simulink model "BS_ur10v"  (R2021b)
settings: Solver=VariableStepAuto  StartTime=0.0  StopTime=15.0  RelTol=1e-3
undefined symbols (not defined in the file): Kd, l1, l2, l3, l4, l5, l6, lambda, m1, m2, m3, m4, m5, m6, q0, r
libraries: roblocks x3
(part 1 of 3)
settings Model: Creator=pierg  LastModifiedBy=vince

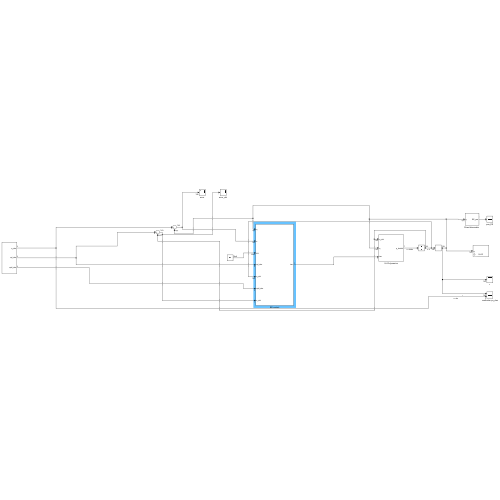
[thumbnail: Simulink's stored preview of the top-level diagram]
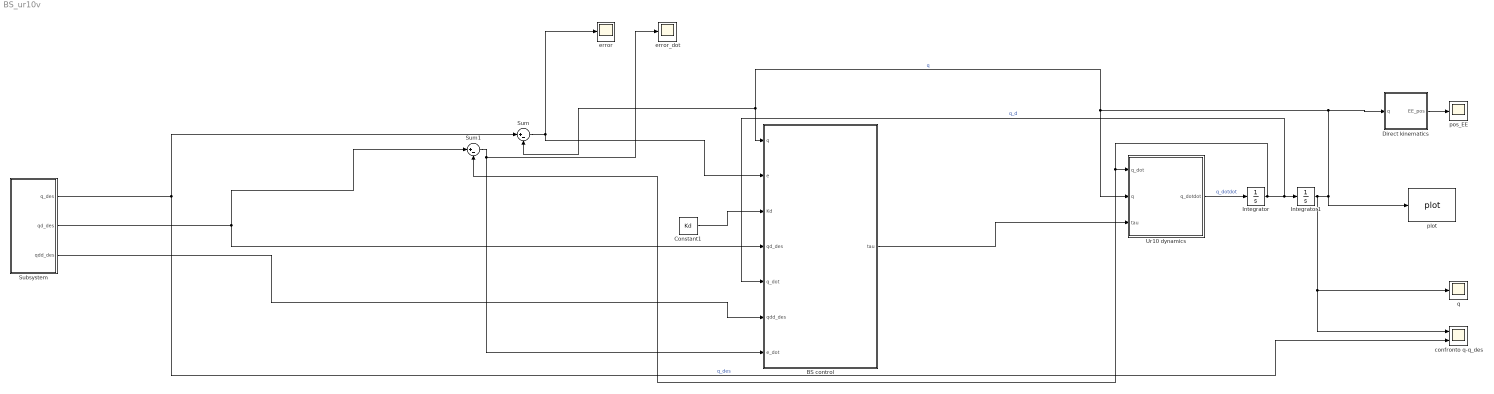
== system BS_ur10v ==
  BS control : Subsystem
  Constant1 : Constant  Value=Kd
  Direct kinematics : Subsystem
  Integrator : Integrator  InitialCondition=[0.001 0.001 0.001 0.001 0.001 0.001]'
  Integrator1 : Integrator  InitialCondition=q0'
  Subsystem : Subsystem
  Sum : Sum  Inputs=|+-
  Sum1 : Sum  Inputs=|+-
  Ur10 dynamics : Subsystem
  confronto q-q_des : Scope  NumInputPorts=2
  error : Scope
  error_dot : Scope
  plot : roblocks/Arm/plot  robot=ur10  fps=20  holdplot=on
  pos_EE : Scope
  q : Scope
  wires:
  Ur10 dynamics/1(q_dotdot) -> Integrator/1  "q_dotdot"
  Integrator/1 -> Ur10 dynamics/1(q_dot), Sum1/2, BS control/5(q_dot), Integrator1/1  "q_d"
  BS control/1(tau) -> Ur10 dynamics/3(tau)
  Integrator1/1 -> confronto q-q_des/1, q/1, plot/1, Direct kinematics/1(q), Ur10 dynamics/2(q), Sum/2, BS control/1(q)  "q"
  Constant1/1 -> BS control/3(Kd)
  Subsystem/1(q_des) -> Sum/1, confronto q-q_des/2  "q_des"
  Subsystem/2(qd_des) -> BS control/4(qd_des), Sum1/1
  Sum/1 -> error/1, BS control/2(e)
  Sum1/1 -> BS control/7(e_dot), error_dot/1
  Direct kinematics/1(EE_pos) -> pos_EE/1
  Subsystem/3(qdd_des) -> BS control/6(qdd_des)

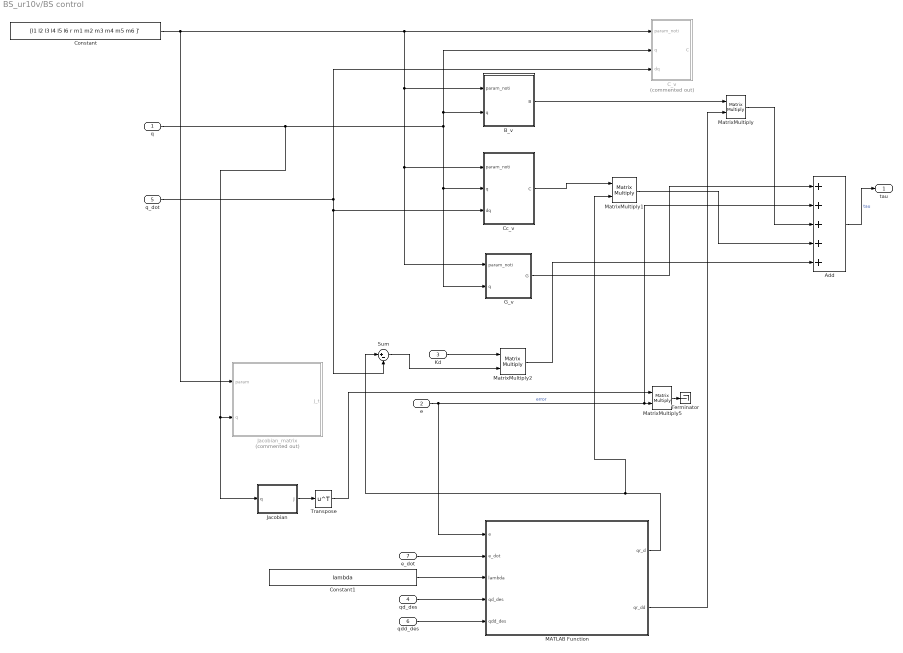
== system BS_ur10v/BS control ==
  q : Inport
  e : Inport  Port=2
  Kd : Inport  Port=3
  qd_des : Inport  Port=4
  q_dot : Inport  Port=5
  qdd_des : Inport  Port=6
  e_dot : Inport  Port=7
  Add : Sum  Inputs=+++++
  B_v : MATLAB Function  TreatAsAtomicUnit=on
  C_v : MATLAB Function  Commented=on  TreatAsAtomicUnit=on
  Cc_v : MATLAB Function  TreatAsAtomicUnit=on
  Constant : Constant  Value=[l1 l2 l3 l4 l5 l6 r m1 m2 m3 m4 m5 m6 ]'
  Constant1 : Constant  Value=lambda
  G_v : MATLAB Function  TreatAsAtomicUnit=on
  Jacobian : MATLAB Function  TreatAsAtomicUnit=on
  Jacobian_matrix : MATLAB Function  Commented=on  TreatAsAtomicUnit=on
  MATLAB Function : MATLAB Function  TreatAsAtomicUnit=on
  MatrixMultiply{,1..2,5} (4 alike) : Product  Multiplication=Matrix(*)
  Sum : Sum  Inputs=|+-
  Terminator : Terminator
  Transpose : Math  Operator=transpose  SaturateOnIntegerOverflow=on
  tau : Outport
  wires:
  Add/1 -> tau/1  "tau"
  B_v/1(B) -> MatrixMultiply/1
  q/1 -> Jacobian_matrix/2(q), Jacobian/1(q), C_v/2(q), B_v/2(q), G_v/2(q), Cc_v/2(q)
  e/1 -> Add/2, MatrixMultiply5/2, MATLAB Function/1(e)  "error"
  MatrixMultiply1/1 -> Add/4
  MatrixMultiply/1 -> Add/3
  G_v/1(G) -> Add/1
  Kd/1 -> MatrixMultiply2/1
  Sum/1 -> MatrixMultiply2/2
  Constant1/1 -> MATLAB Function/3(lambda)
  Constant/1 -> Jacobian_matrix/1(param), G_v/1(param_noti), Cc_v/1(param_noti), B_v/1(param_noti), C_v/1(param_noti)
  qd_des/1 -> MATLAB Function/4(qd_des)
  MATLAB Function/1(qr_d) -> Sum/1, MatrixMultiply1/2
  q_dot/1 -> Sum/2, Cc_v/3(dq), C_v/3(dq)
  MatrixMultiply2/1 -> Add/5
  qdd_des/1 -> MATLAB Function/5(qdd_des)
  e_dot/1 -> MATLAB Function/2(e_dot)
  MATLAB Function/2(qr_dd) -> MatrixMultiply/2
  Jacobian/1(J) -> Transpose/1
  Transpose/1 -> MatrixMultiply5/1
  Cc_v/1(C) -> MatrixMultiply1/1
  MatrixMultiply5/1 -> Terminator/1

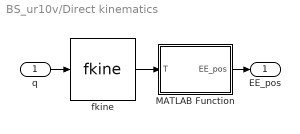
== system BS_ur10v/Direct kinematics ==
  q : Inport
  MATLAB Function : MATLAB Function  TreatAsAtomicUnit=on
  fkine : roblocks/Arm/fkine  robot=ur10
  EE_pos : Outport
  wires:
  q/1 -> fkine/1
  MATLAB Function/1(EE_pos) -> EE_pos/1
  fkine/1 -> MATLAB Function/1(T)

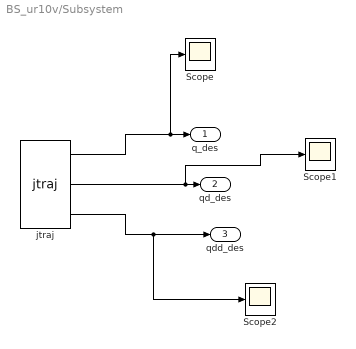
== system BS_ur10v/Subsystem ==
  Scope : Scope
  Scope1 : Scope
  Scope2 : Scope
  jtraj : roblocks/Toolbox/jtraj  q0=q0  qf=q_des_fin  tmax=15  ts=0.1
  q_des : Outport
  qd_des : Outport  Port=2
  qdd_des : Outport  Port=3
  wires:
  jtraj/2 -> Scope1/1, qd_des/1
  jtraj/3 -> qdd_des/1, Scope2/1
  jtraj/1 -> Scope/1, q_des/1

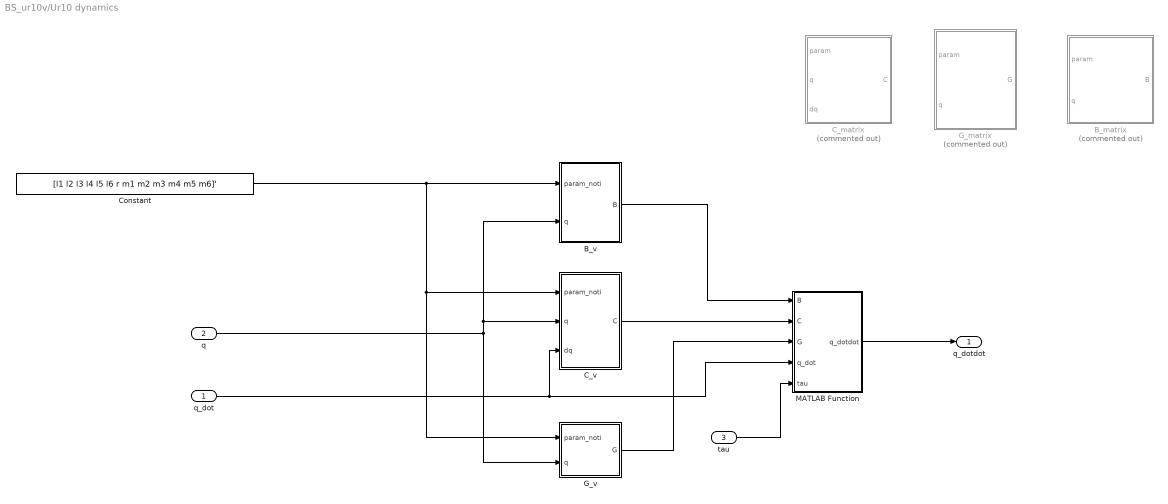
== system BS_ur10v/Ur10 dynamics ==
  q_dot : Inport
  q : Inport  Port=2
  tau : Inport  Port=3
  B_matrix : MATLAB Function  Commented=on  TreatAsAtomicUnit=on
  B_v : MATLAB Function  TreatAsAtomicUnit=on
  C_matrix : MATLAB Function  Commented=on  TreatAsAtomicUnit=on
  C_v : MATLAB Function  TreatAsAtomicUnit=on
  Constant : Constant  Value=[l1 l2 l3 l4 l5 l6 r m1 m2 m3 m4 m5 m6]'
  G_matrix : MATLAB Function  Commented=on  TreatAsAtomicUnit=on
  G_v : MATLAB Function  TreatAsAtomicUnit=on
  MATLAB Function : MATLAB Function  TreatAsAtomicUnit=on
  q_dotdot : Outport
  wires:
  Constant/1 -> G_v/1(param_noti), C_v/1(param_noti), B_v/1(param_noti)
  q/1 -> B_v/2(q), C_v/2(q), G_v/2(q)
  MATLAB Function/1(q_dotdot) -> q_dotdot/1
  q_dot/1 -> C_v/3(dq), MATLAB Function/4(q_dot)
  tau/1 -> MATLAB Function/5(tau)
  B_v/1(B) -> MATLAB Function/1(B)
  C_v/1(C) -> MATLAB Function/2(C)
  G_v/1(G) -> MATLAB Function/3(G)

== matlab function BS_ur10v/Ur10 dynamics/MATLAB Function ==
  data: B input; q_dotdot output; C input; G input; q_dot input; tau input
function q_dotdot = dynamics(B, C, G, q_dot, tau)
% Calcolo l'accelerazione dei giunti
q_dotdot = B \ (tau - C*q_dot - G);

== matlab function BS_ur10v/BS control/Jacobian ==
  data: q input; J output
function J = Jacobian(q)

q1 = q(1);
q2 = q(2);
q3 = q(3);
q4 = q(4);
q5 = q(5);
q6 = q(6);
%#codegen

%    This function was generated by the Symbolic Math Toolbox version 9.0.
%    01-Oct-2022 19:35:43

t2 = cos(q1);
t3 = cos(q2);
t4 = cos(q3);
t5 = cos(q4);
t6 = cos(q5);
t7 = sin(q1);
t8 = sin(q2);
t9 = sin(q3);
t10 = sin(q4);
t11 = sin(q5);
t12 = q2+q3;
t16 = -q5;
t13 = cos(t12);
t14 = q4+t12;
t15 = sin(t12);
t20 = -t2;
t24 = t8.*(1.53e+2./2.5e+2);
t17 = cos(t14);
t18 = q5+t14;
t19 = sin(t14);
t22 = t14+t16;
t25 = t13.*5.723e-1;
t26 = t15.*5.723e-1;
t27 = t10.*t13.*9.22e-2;
t28 = t5.*t15.*9.22e-2;
t34 = t5.*t13.*1.157e-1;
t36 = t10.*t15.*1.157e-1;
t21 = sin(t18);
t23 = sin(t22);
t29 = -t25;
t30 = t11.*t19.*9.22e-2;
t31 = t17.*1.157e-1;
t32 = t19.*1.157e-1;
t37 = -t36;
t39 = t27+t28;
t33 = t21.*4.61e-2;
t38 = t23.*4.61e-2;
t40 = t30+t31;
t41 = t11.*t39;
t35 = -t33;
t42 = t26+t40;
t43 = t24+t26+t34+t37+t41;
mt1 = [t2.*1.639e-1+t2.*t6.*9.22e-2+t3.*t7.*(1.53e+2./2.5e+2)+t3.*t4.*t7.*5.723e-1-t7.*t8.*t9.*5.723e-1-t5.*t7.*t15.*1.157e-1-t7.*t10.*t13.*1.157e-1+t7.*t11.*t17.*9.22e-2];
mt2 = [t7.*1.639e-1-t2.*t3.*(1.53e+2./2.5e+2)+t6.*t7.*9.22e-2-t2.*t3.*t4.*5.723e-1+t2.*t8.*t9.*5.723e-1+t2.*t5.*t15.*1.157e-1+t2.*t10.*t13.*1.157e-1-t2.*t11.*t17.*9.22e-2,0.0,0.0,0.0,1.0,t2.*t43,t7.*t43,t3.*(-1.53e+2./2.5e+2)+t29+t32+t35+t38,t7,t20,0.0,t2.*t42,t7.*t42,t29+t32+t35+t38,t7,t20,0.0,t2.*t40,t7.*t40,t32+t35+t38,t7,t20,0.0];
mt3 = [t7.*t11.*(-9.22e-2)-t2.*t3.*t4.*t5.*t6.*9.22e-2+t2.*t3.*t6.*t9.*t10.*9.22e-2+t2.*t4.*t6.*t8.*t10.*9.22e-2+t2.*t5.*t6.*t8.*t9.*9.22e-2,t2.*t11.*9.22e-2-t3.*t4.*t5.*t6.*t7.*9.22e-2+t3.*t6.*t7.*t9.*t10.*9.22e-2+t4.*t6.*t7.*t8.*t10.*9.22e-2+t5.*t6.*t7.*t8.*t9.*9.22e-2,t35-t38,t2.*t19,t7.*t19,-t17,0.0,0.0,0.0,t6.*t7+t11.*t17.*t20,t6.*t20-t7.*t11.*t17,-t11.*t19];
J = reshape([mt1,mt2,mt3],6,6);

== matlab function BS_ur10v/BS control/MATLAB Function ==
  data: e input; qr_d output; e_dot input; lambda input; qd_des input; qdd_des input; qr_dd output
function [qr_d , qr_dd]= qr_d_calculus(e,e_dot,lambda,qd_des,qdd_des)

qr_d = qd_des + lambda*e;

qr_dd = qdd_des + lambda*e_dot;


end

== matlab function BS_ur10v/Ur10 dynamics/C_v ==
  data: param_noti input; C output; q input; dq input
function C = C_v(param_noti, q, dq)
%#codegen
l1 = param_noti(1);
l2 = param_noti(2);
l3 = param_noti(3);
l4 = param_noti(4);
l5 = param_noti(5);
l6 = param_noti(6);
r  = param_noti(7);

m1 = param_noti(8);
m2 = param_noti(9);
m3 = param_noti(10);
m4 = param_noti(11);
m5 = param_noti(12);
m6 = param_noti(13);


q1 = q(1);
q2 = q(2);
q3 = q(3);
q4 = q(4);
q5 = q(5);
q6 = q(6);

dq1 = dq(1);
dq2 = dq(2);
dq3 = dq(3);
dq4 = dq(4);
dq5 = dq(5);
dq6 = dq(6);

%    This function was generated by the Symbolic Math Toolbox version 9.0.
%    24-Sep-2022 17:47:23

t2 = cos(q2);
t3 = cos(q3);
t4 = cos(q4);
t5 = cos(q5);
t6 = sin(q3);
t7 = sin(q4);
t8 = sin(q5);
t9 = q2+q3;
t10 = q2+q5;
t11 = q3+q4;
t12 = q4+q5;
t13 = l2.^2;
t14 = l3.^2;
t15 = l4.^2;
t16 = l5.^2;
t17 = l6.^2;
t18 = q2.*2.0;
t19 = q3.*2.0;
t20 = q4.*2.0;
t21 = q5.*2.0;
t22 = r.^2;
t32 = -q5;
t23 = sin(t18);
t24 = sin(t21);
t25 = cos(t9);
t26 = cos(t10);
t27 = cos(t11);
t28 = cos(t12);
t29 = q4+t9;
t30 = q5+t9;
t31 = q5+t11;
t33 = -t21;
t36 = t9+t12;
t38 = q2+t9;
t42 = q2+t32;
t43 = q4+t32;
t44 = t9.*2.0;
t47 = t9+t32;
t48 = t11+t32;
t50 = l3.*l5.*m6.*t4.*2.0;
t53 = dq2.*l3.*l5.*m6.*t4;
t54 = dq3.*l3.*l5.*m6.*t4;
t55 = dq4.*l3.*l5.*m6.*t4;
t56 = dq2.*l2.*l3.*m3.*t6;
t57 = dq2.*l2.*l3.*m4.*t6;
t58 = dq2.*l2.*l3.*m6.*t6;
t59 = dq1.*l4.*l6.*m6.*t8;
t60 = dq5.*l5.*l6.*m6.*t8;
t69 = l2.*l5.*m6.*t3.*t4.*2.0;
t70 = l3.*l6.*m6.*t4.*t5.*2.0;
t71 = l2.*l5.*m6.*t6.*t7.*2.0;
t72 = l3.*l6.*m6.*t7.*t8.*2.0;
t77 = dq2.*l2.*l5.*m6.*t3.*t4;
t78 = dq5.*l3.*l6.*m6.*t4.*t5;
t79 = dq2.*l2.*l5.*m6.*t6.*t7;
t80 = dq2.*l3.*l6.*m6.*t7.*t8;
t81 = dq3.*l3.*l6.*m6.*t7.*t8;
t82 = dq4.*l3.*l6.*m6.*t7.*t8;
t94 = (dq1.*l3.*l5.*m6.*t4)./2.0;
t96 = (dq1.*l2.*l3.*m3.*t6)./2.0;
t97 = (dq1.*l2.*l3.*m4.*t6)./2.0;
t98 = (dq1.*l2.*l3.*m6.*t6)./2.0;
t102 = l2.*l6.*m6.*t3.*t7.*t8.*2.0;
t103 = l2.*l6.*m6.*t4.*t6.*t8.*2.0;
t107 = dq2.*l2.*l6.*m6.*t3.*t7.*t8;
t108 = dq2.*l2.*l6.*m6.*t4.*t6.*t8;
t117 = (dq2.*m6.*t8.*t22)./4.0;
t118 = (dq3.*m6.*t8.*t22)./4.0;
t119 = (dq4.*m6.*t8.*t22)./4.0;
t120 = (dq5.*m6.*t8.*t22)./4.0;
t121 = (dq6.*m6.*t8.*t22)./4.0;
t126 = (m5.*t5.*t8.*t16)./6.0;
t128 = (m5.*t5.*t8.*t22)./2.0;
t129 = (m6.*t5.*t8.*t22)./2.0;
t157 = m6.*t5.*t8.*t17.*(1.3e+1./6.0);
t34 = cos(t30);
t35 = cos(t31);
t37 = sin(t29);
t39 = q2+t29;
t40 = sin(t38);
t41 = sin(t36);
t45 = cos(t42);
t46 = cos(t43);
t51 = t12+t30;
t52 = t10+t29;
t61 = t9+t29;
t62 = sin(t44);
t63 = cos(t47);
t64 = cos(t48);
t65 = t29+t32;
t66 = t29+t33;
t73 = dq2.*l3.*l4.*m4.*t25;
t74 = dq3.*l3.*l4.*m4.*t25;
t75 = dq2.*l3.*l4.*m6.*t25;
t76 = dq3.*l3.*l4.*m6.*t25;
t84 = -t53;
t85 = -t54;
t86 = t9+t36;
t93 = t20+t44;
t104 = t29+t36;
t113 = -t77;
t114 = -t78;
t115 = -t80;
t116 = -t81;
t125 = t29+t47;
t131 = (dq1.*l2.*l5.*m6.*t27)./2.0;
t132 = (dq1.*l2.*l6.*m6.*t26)./2.0;
t133 = (dq2.*l2.*l6.*m6.*t26)./2.0;
t134 = (dq2.*l3.*l6.*m6.*t28)./2.0;
t135 = (dq5.*l2.*l6.*m6.*t26)./2.0;
t136 = (dq1.*l3.*l6.*m6.*t28)./4.0;
t137 = (dq3.*l3.*l6.*m6.*t28)./2.0;
t138 = (dq4.*l3.*l6.*m6.*t28)./2.0;
t139 = (dq5.*l3.*l6.*m6.*t28)./2.0;
t141 = -t120;
t142 = -t121;
t152 = (dq1.*m2.*t13.*t23)./2.0;
t153 = (dq1.*m3.*t13.*t23)./2.0;
t154 = (dq1.*m4.*t13.*t23)./2.0;
t155 = (dq1.*m6.*t13.*t23)./2.0;
t156 = -t126;
t158 = t36.*2.0;
t160 = -t107;
t161 = -t108;
t181 = (dq2.*m5.*t16.*t24)./2.4e+1;
t182 = (dq3.*m5.*t16.*t24)./2.4e+1;
t183 = (dq4.*m5.*t16.*t24)./2.4e+1;
t184 = (dq5.*m5.*t16.*t24)./2.4e+1;
t185 = (dq1.*m5.*t16.*t24)./4.8e+1;
t186 = (dq2.*m5.*t22.*t24)./8.0;
t187 = (dq2.*m6.*t22.*t24)./8.0;
t188 = (dq3.*m5.*t22.*t24)./8.0;
t189 = (dq3.*m6.*t22.*t24)./8.0;
t190 = (dq4.*m5.*t22.*t24)./8.0;
t191 = (dq4.*m6.*t22.*t24)./8.0;
t192 = (dq5.*m5.*t22.*t24)./8.0;
t193 = (dq5.*m6.*t22.*t24)./8.0;
t194 = (dq1.*m5.*t22.*t24)./1.6e+1;
t195 = (dq1.*m6.*t22.*t24)./1.6e+1;
t196 = -t157;
t237 = dq2.*m6.*t17.*t24.*(1.3e+1./2.4e+1);
t238 = dq3.*m6.*t17.*t24.*(1.3e+1./2.4e+1);
t239 = dq4.*m6.*t17.*t24.*(1.3e+1./2.4e+1);
t240 = dq5.*m6.*t17.*t24.*(1.3e+1./2.4e+1);
t241 = dq1.*m6.*t17.*t24.*(1.3e+1./4.8e+1);
t49 = cos(t39);
t67 = cos(t52);
t68 = sin(t51);
t83 = cos(t61);
t87 = sin(t65);
t88 = sin(t66);
t89 = dq2.*l4.*l5.*m6.*t37;
t90 = dq3.*l4.*l5.*m6.*t37;
t91 = dq4.*l4.*l5.*m6.*t37;
t92 = cos(t86);
t95 = t32+t39;
t99 = dq1.*l2.*l3.*m3.*t40;
t100 = dq1.*l2.*l3.*m4.*t40;
t101 = dq1.*l2.*l3.*m6.*t40;
t105 = sin(t93);
t109 = -t73;
t110 = -t74;
t111 = -t75;
t112 = -t76;
t140 = sin(t104);
t143 = (dq1.*l3.*l6.*m6.*t34)./2.0;
t144 = (dq2.*l3.*l6.*m6.*t34)./2.0;
t145 = (dq2.*l2.*l6.*m6.*t35)./2.0;
t146 = (dq3.*l3.*l6.*m6.*t34)./2.0;
t147 = (dq1.*l2.*l6.*m6.*t35)./4.0;
t148 = (dq3.*l2.*l6.*m6.*t35)./2.0;
t149 = (dq4.*l2.*l6.*m6.*t35)./2.0;
t150 = (dq5.*l3.*l6.*m6.*t34)./2.0;
t151 = (dq5.*l2.*l6.*m6.*t35)./2.0;
t159 = cos(t125);
t162 = -t131;
t163 = -t134;
t164 = -t136;
t165 = -t137;
t166 = -t138;
t167 = -t139;
t168 = sin(t158);
t197 = (dq1.*l5.*l6.*m6.*t41)./2.0;
t198 = (dq2.*l4.*l6.*m6.*t41)./2.0;
t199 = (dq2.*l5.*l6.*m6.*t41)./2.0;
t200 = (dq3.*l4.*l6.*m6.*t41)./2.0;
t201 = (dq3.*l5.*l6.*m6.*t41)./2.0;
t202 = (dq4.*l4.*l6.*m6.*t41)./2.0;
t203 = (dq4.*l5.*l6.*m6.*t41)./2.0;
t204 = (dq5.*l4.*l6.*m6.*t41)./2.0;
t205 = (dq5.*l5.*l6.*m6.*t41)./2.0;
t206 = t32+t93;
t207 = t33+t93;
t209 = (dq1.*l2.*l6.*m6.*t45)./2.0;
t210 = (dq2.*l2.*l6.*m6.*t45)./2.0;
t211 = (dq2.*l3.*l6.*m6.*t46)./2.0;
t212 = (dq5.*l2.*l6.*m6.*t45)./2.0;
t213 = (dq1.*l3.*l6.*m6.*t46)./4.0;
t214 = (dq3.*l3.*l6.*m6.*t46)./2.0;
t215 = (dq4.*l3.*l6.*m6.*t46)./2.0;
t216 = (dq5.*l3.*l6.*m6.*t46)./2.0;
t219 = (dq1.*m5.*t16.*t37)./2.4e+1;
t220 = (dq2.*m5.*t16.*t37)./2.4e+1;
t221 = (dq3.*m5.*t16.*t37)./2.4e+1;
t222 = (dq4.*m5.*t16.*t37)./2.4e+1;
t223 = (dq5.*m5.*t16.*t37)./2.4e+1;
t224 = (dq1.*m5.*t22.*t37)./8.0;
t225 = (dq1.*m6.*t22.*t37)./8.0;
t226 = (dq2.*m5.*t22.*t37)./8.0;
t227 = (dq2.*m6.*t22.*t37)./8.0;
t228 = (dq3.*m5.*t22.*t37)./8.0;
t229 = (dq3.*m6.*t22.*t37)./8.0;
t230 = (dq4.*m5.*t22.*t37)./8.0;
t231 = (dq4.*m6.*t22.*t37)./8.0;
t232 = (dq5.*m5.*t22.*t37)./8.0;
t233 = (dq5.*m6.*t22.*t37)./8.0;
t234 = -t181;
t235 = -t182;
t236 = -t183;
t242 = -t186;
t243 = -t187;
t244 = -t188;
t245 = -t189;
t246 = -t190;
t247 = -t191;
t248 = -t192;
t249 = -t193;
t263 = dq1.*m6.*t17.*t37.*(1.3e+1./2.4e+1);
t264 = dq2.*m6.*t17.*t37.*(1.3e+1./2.4e+1);
t265 = dq3.*m6.*t17.*t37.*(1.3e+1./2.4e+1);
t266 = dq4.*m6.*t17.*t37.*(1.3e+1./2.4e+1);
t267 = dq5.*m6.*t17.*t37.*(1.3e+1./2.4e+1);
t272 = -t237;
t273 = -t238;
t274 = -t239;
t276 = (dq1.*l3.*l6.*m6.*t63)./2.0;
t277 = (dq2.*l3.*l6.*m6.*t63)./2.0;
t278 = (dq2.*l2.*l6.*m6.*t64)./2.0;
t279 = (dq3.*l3.*l6.*m6.*t63)./2.0;
t280 = (dq1.*l2.*l6.*m6.*t64)./4.0;
t281 = (dq3.*l2.*l6.*m6.*t64)./2.0;
t282 = (dq4.*l2.*l6.*m6.*t64)./2.0;
t283 = (dq5.*l3.*l6.*m6.*t63)./2.0;
t284 = (dq5.*l2.*l6.*m6.*t64)./2.0;
t285 = (dq6.*m6.*t22.*t41)./8.0;
t292 = (dq1.*m3.*t14.*t62)./2.0;
t293 = (dq1.*m4.*t14.*t62)./2.0;
t294 = (dq1.*m6.*t14.*t62)./2.0;
t106 = cos(t95);
t122 = -t89;
t123 = -t90;
t124 = -t91;
t127 = -t87;
t130 = dq1.*l2.*l5.*m6.*t49;
t169 = t99./2.0;
t170 = t100./2.0;
t171 = t101./2.0;
t172 = -t143;
t173 = -t144;
t174 = -t145;
t175 = -t146;
t176 = -t147;
t177 = -t148;
t178 = -t149;
t179 = -t150;
t180 = -t151;
t208 = dq1.*l3.*l5.*m6.*t83;
t217 = sin(t206);
t218 = sin(t207);
t251 = -t197;
t252 = -t199;
t253 = -t201;
t254 = -t203;
t255 = -t205;
t256 = -t210;
t257 = -t211;
t258 = -t213;
t259 = -t214;
t260 = -t215;
t261 = -t219;
t262 = -t223;
t268 = -t224;
t269 = -t225;
t270 = -t232;
t271 = -t233;
t287 = t41+t87;
t288 = (dq1.*l2.*l6.*m6.*t67)./2.0;
t289 = (dq1.*l2.*l6.*m6.*t67)./4.0;
t290 = -t263;
t291 = -t267;
t295 = -t276;
t296 = -t277;
t297 = -t279;
t298 = -t280;
t299 = -t285;
t302 = (dq1.*l5.*l6.*m6.*t87)./2.0;
t303 = (dq2.*l4.*l6.*m6.*t87)./2.0;
t304 = (dq2.*l5.*l6.*m6.*t87)./2.0;
t305 = (dq3.*l4.*l6.*m6.*t87)./2.0;
t306 = (dq3.*l5.*l6.*m6.*t87)./2.0;
t307 = (dq4.*l4.*l6.*m6.*t87)./2.0;
t308 = (dq4.*l5.*l6.*m6.*t87)./2.0;
t309 = (dq5.*l4.*l6.*m6.*t87)./2.0;
t310 = (dq5.*l5.*l6.*m6.*t87)./2.0;
t311 = (dq1.*l3.*l6.*m6.*t92)./2.0;
t312 = (dq1.*l3.*l6.*m6.*t92)./4.0;
t313 = -t292;
t314 = -t293;
t315 = -t294;
t316 = (dq1.*m5.*t16.*t68)./4.8e+1;
t317 = (dq2.*m5.*t16.*t68)./4.8e+1;
t318 = (dq3.*m5.*t16.*t68)./4.8e+1;
t319 = (dq4.*m5.*t16.*t68)./4.8e+1;
t320 = (dq5.*m5.*t16.*t68)./4.8e+1;
t321 = (dq1.*m5.*t22.*t68)./1.6e+1;
t322 = (dq1.*m6.*t22.*t68)./1.6e+1;
t323 = (dq2.*m5.*t22.*t68)./1.6e+1;
t324 = (dq2.*m6.*t22.*t68)./1.6e+1;
t325 = (dq3.*m5.*t22.*t68)./1.6e+1;
t326 = (dq3.*m6.*t22.*t68)./1.6e+1;
t327 = (dq4.*m5.*t22.*t68)./1.6e+1;
t328 = (dq4.*m6.*t22.*t68)./1.6e+1;
t329 = (dq5.*m5.*t22.*t68)./1.6e+1;
t330 = (dq5.*m6.*t22.*t68)./1.6e+1;
t343 = (dq1.*m5.*t16.*t88)./4.8e+1;
t345 = (dq2.*m5.*t16.*t88)./4.8e+1;
t346 = (dq3.*m5.*t16.*t88)./4.8e+1;
t347 = (dq4.*m5.*t16.*t88)./4.8e+1;
t348 = (dq5.*m5.*t16.*t88)./4.8e+1;
t349 = dq1.*m6.*t17.*t68.*(1.3e+1./4.8e+1);
t350 = dq2.*m6.*t17.*t68.*(1.3e+1./4.8e+1);
t351 = dq3.*m6.*t17.*t68.*(1.3e+1./4.8e+1);
t352 = dq4.*m6.*t17.*t68.*(1.3e+1./4.8e+1);
t353 = dq5.*m6.*t17.*t68.*(1.3e+1./4.8e+1);
t354 = (dq6.*m6.*t22.*t87)./8.0;
t355 = (dq1.*m5.*t22.*t88)./1.6e+1;
t357 = (dq1.*m6.*t22.*t88)./1.6e+1;
t359 = (dq2.*m5.*t22.*t88)./1.6e+1;
t361 = (dq2.*m6.*t22.*t88)./1.6e+1;
t363 = (dq3.*m5.*t22.*t88)./1.6e+1;
t365 = (dq3.*m6.*t22.*t88)./1.6e+1;
t367 = (dq4.*m5.*t22.*t88)./1.6e+1;
t369 = (dq4.*m6.*t22.*t88)./1.6e+1;
t371 = (dq5.*m5.*t22.*t88)./1.6e+1;
t373 = (dq5.*m6.*t22.*t88)./1.6e+1;
t375 = (dq1.*m6.*t16.*t105)./2.0;
t377 = (dq1.*l5.*l6.*m6.*t140)./2.0;
t378 = (dq1.*l5.*l6.*m6.*t140)./4.0;
t383 = dq1.*m6.*t17.*t88.*(1.3e+1./4.8e+1);
t385 = dq2.*m6.*t17.*t88.*(1.3e+1./4.8e+1);
t386 = dq3.*m6.*t17.*t88.*(1.3e+1./4.8e+1);
t387 = dq4.*m6.*t17.*t88.*(1.3e+1./4.8e+1);
t388 = dq5.*m6.*t17.*t88.*(1.3e+1./4.8e+1);
t395 = (dq1.*m4.*t15.*t105)./2.4e+1;
t396 = (dq1.*m5.*t16.*t105)./4.8e+1;
t397 = (dq1.*m4.*t22.*t105)./8.0;
t398 = (dq1.*m5.*t22.*t105)./1.6e+1;
t399 = (dq1.*m6.*t22.*t105)./1.6e+1;
t400 = (dq1.*l3.*l6.*m6.*t159)./2.0;
t401 = (dq1.*l3.*l6.*m6.*t159)./4.0;
t409 = dq1.*m6.*t17.*t105.*(1.3e+1./4.8e+1);
t418 = (dq1.*m5.*t22.*t168)./3.2e+1;
t419 = (dq1.*m6.*t22.*t168)./3.2e+1;
t421 = (dq1.*m5.*t16.*t168)./9.6e+1;
t428 = dq1.*m6.*t17.*t168.*(1.3e+1./9.6e+1);
t250 = t130./2.0;
t286 = -t208;
t300 = t208./2.0;
t301 = -t289;
t331 = -t302;
t332 = -t303;
t333 = -t304;
t334 = -t305;
t335 = -t306;
t336 = -t307;
t337 = -t308;
t338 = t41+t127;
t339 = (dq1.*l2.*l6.*m6.*t106)./2.0;
t340 = (dq1.*l2.*l6.*m6.*t106)./4.0;
t341 = -t311;
t342 = -t312;
t344 = -t316;
t356 = -t321;
t358 = -t322;
t360 = -t323;
t362 = -t324;
t364 = -t325;
t366 = -t326;
t368 = -t327;
t370 = -t328;
t372 = -t329;
t374 = -t330;
t379 = -t343;
t380 = -t345;
t381 = -t346;
t382 = -t347;
t384 = -t349;
t389 = -t354;
t390 = -t355;
t391 = -t357;
t392 = -t371;
t393 = -t373;
t394 = -t375;
t402 = -t377;
t403 = -t383;
t404 = -t385;
t405 = -t386;
t406 = -t387;
t407 = -t395;
t408 = -t396;
t410 = -t397;
t411 = -t398;
t412 = -t399;
t413 = -t400;
t414 = -t401;
t415 = (dq1.*l5.*l6.*m6.*t217)./2.0;
t416 = (dq1.*l5.*l6.*m6.*t217)./4.0;
t417 = -t409;
t422 = (dq1.*m5.*t22.*t218)./3.2e+1;
t423 = -t418;
t424 = (dq1.*m6.*t22.*t218)./3.2e+1;
t425 = -t419;
t426 = (dq1.*m5.*t16.*t218)./9.6e+1;
t427 = -t421;
t431 = (dq1.*m6.*t22.*t287)./8.0;
t432 = (dq5.*m6.*t22.*t287)./8.0;
t434 = dq1.*m6.*t17.*t218.*(1.3e+1./9.6e+1);
t435 = -t428;
t275 = -t250;
t376 = -t340;
t420 = -t415;
t429 = -t422;
t430 = -t424;
t433 = -t426;
t436 = -t432;
t437 = -t434;
t438 = (dq1.*m6.*t22.*t338)./8.0;
t439 = (dq2.*m6.*t22.*t338)./8.0;
t440 = (dq3.*m6.*t22.*t338)./8.0;
t441 = (dq4.*m6.*t22.*t338)./8.0;
t442 = -t438;
t443 = -t439;
t444 = -t440;
t445 = -t441;
t446 = t141+t438;
t447 = t141+t442;
t448 = t436+t443+t444+t445;
et1 = t55./2.0-(dq2.*m2.*t13.*t23)./2.0-(dq2.*m3.*t13.*t23)./2.0-(dq2.*m4.*t13.*t23)./2.0-(dq2.*m6.*t13.*t23)./2.0-(dq5.*m5.*t16.*t24)./4.8e+1-dq5.*m6.*t17.*t24.*(1.3e+1./4.8e+1)+(dq5.*m5.*t22.*t24)./1.6e+1+(dq5.*m6.*t22.*t24)./1.6e+1-(dq2.*m3.*t14.*t62)./2.0-(dq2.*m4.*t14.*t62)./2.0-(dq3.*m3.*t14.*t62)./2.0-(dq3.*m4.*t14.*t62)./2.0-(dq2.*m6.*t14.*t62)./2.0-(dq3.*m6.*t14.*t62)./2.0+(dq2.*m4.*t15.*t105)./2.4e+1+(dq3.*m4.*t15.*t105)./2.4e+1-(dq2.*m5.*t16.*t105)./4.8e+1+(dq4.*m4.*t15.*t105)./2.4e+1+(dq2.*m6.*t16.*t105)./2.0-(dq3.*m5.*t16.*t105)./4.8e+1-dq2.*m6.*t17.*t105.*(1.3e+1./4.8e+1);
et2 = (dq3.*m6.*t16.*t105)./2.0-(dq4.*m5.*t16.*t105)./4.8e+1-dq3.*m6.*t17.*t105.*(1.3e+1./4.8e+1)+(dq4.*m6.*t16.*t105)./2.0-dq4.*m6.*t17.*t105.*(1.3e+1./4.8e+1)-(dq2.*m4.*t22.*t105)./8.0+(dq2.*m5.*t22.*t105)./1.6e+1-(dq3.*m4.*t22.*t105)./8.0+(dq2.*m6.*t22.*t105)./1.6e+1+(dq3.*m5.*t22.*t105)./1.6e+1-(dq4.*m4.*t22.*t105)./8.0+(dq3.*m6.*t22.*t105)./1.6e+1+(dq4.*m5.*t22.*t105)./1.6e+1+(dq4.*m6.*t22.*t105)./1.6e+1+(dq2.*m5.*t16.*t168)./9.6e+1+(dq3.*m5.*t16.*t168)./9.6e+1+dq2.*m6.*t17.*t168.*(1.3e+1./9.6e+1)+(dq4.*m5.*t16.*t168)./9.6e+1+dq3.*m6.*t17.*t168.*(1.3e+1./9.6e+1)+(dq5.*m5.*t16.*t168)./9.6e+1;
et3 = dq4.*m6.*t17.*t168.*(1.3e+1./9.6e+1)+dq5.*m6.*t17.*t168.*(1.3e+1./9.6e+1)-(dq2.*m5.*t22.*t168)./3.2e+1-(dq2.*m6.*t22.*t168)./3.2e+1-(dq3.*m5.*t22.*t168)./3.2e+1-(dq3.*m6.*t22.*t168)./3.2e+1-(dq4.*m5.*t22.*t168)./3.2e+1-(dq4.*m6.*t22.*t168)./3.2e+1-(dq5.*m5.*t22.*t168)./3.2e+1-(dq5.*m6.*t22.*t168)./3.2e+1+(dq2.*m5.*t16.*t218)./9.6e+1+(dq3.*m5.*t16.*t218)./9.6e+1+dq2.*m6.*t17.*t218.*(1.3e+1./9.6e+1)+(dq4.*m5.*t16.*t218)./9.6e+1+dq3.*m6.*t17.*t218.*(1.3e+1./9.6e+1)-(dq5.*m5.*t16.*t218)./9.6e+1+dq4.*m6.*t17.*t218.*(1.3e+1./9.6e+1)-dq5.*m6.*t17.*t218.*(1.3e+1./9.6e+1)-(dq2.*m5.*t22.*t218)./3.2e+1;
et4 = dq2.*m6.*t22.*t218.*(-1.0./3.2e+1)-(dq3.*m5.*t22.*t218)./3.2e+1-(dq3.*m6.*t22.*t218)./3.2e+1-(dq4.*m5.*t22.*t218)./3.2e+1-(dq4.*m6.*t22.*t218)./3.2e+1+(dq5.*m5.*t22.*t218)./3.2e+1+(dq5.*m6.*t22.*t218)./3.2e+1-(dq3.*l2.*l3.*m3.*t6)./2.0-(dq3.*l2.*l3.*m4.*t6)./2.0-(dq3.*l2.*l3.*m6.*t6)./2.0-dq5.*l4.*l6.*m6.*t8+(dq3.*l2.*l5.*m6.*t27)./2.0+(dq4.*l2.*l5.*m6.*t27)./2.0-(dq4.*l3.*l6.*m6.*t28)./4.0-(dq5.*l3.*l6.*m6.*t28)./4.0-dq2.*l2.*l3.*m3.*t40-dq2.*l2.*l3.*m4.*t40-(dq3.*l2.*l3.*m3.*t40)./2.0-(dq3.*l2.*l3.*m4.*t40)./2.0-(dq3.*l2.*l6.*m6.*t35)./4.0-dq2.*l2.*l3.*m6.*t40;
et5 = dq4.*l2.*l6.*m6.*t35.*(-1.0./4.0)-(dq3.*l2.*l3.*m6.*t40)./2.0-(dq5.*l2.*l6.*m6.*t35)./4.0+dq2.*l2.*l5.*m6.*t49+(dq3.*l2.*l5.*m6.*t49)./2.0+(dq4.*l3.*l6.*m6.*t46)./4.0+(dq4.*l2.*l5.*m6.*t49)./2.0-(dq5.*l3.*l6.*m6.*t46)./4.0+(dq3.*l2.*l6.*m6.*t64)./4.0+(dq4.*l2.*l6.*m6.*t64)./4.0-(dq2.*l2.*l6.*m6.*t67)./2.0-(dq5.*l2.*l6.*m6.*t64)./4.0-(dq3.*l2.*l6.*m6.*t67)./4.0-(dq4.*l2.*l6.*m6.*t67)./4.0-(dq5.*l2.*l6.*m6.*t67)./4.0+dq2.*l3.*l5.*m6.*t83+dq3.*l3.*l5.*m6.*t83+(dq4.*l3.*l5.*m6.*t83)./2.0-(dq2.*l3.*l6.*m6.*t92)./2.0-(dq3.*l3.*l6.*m6.*t92)./2.0-(dq4.*l3.*l6.*m6.*t92)./4.0;
et6 = dq5.*l3.*l6.*m6.*t92.*(-1.0./4.0)+(dq2.*l2.*l6.*m6.*t106)./2.0+(dq3.*l2.*l6.*m6.*t106)./4.0+(dq4.*l2.*l6.*m6.*t106)./4.0-(dq5.*l2.*l6.*m6.*t106)./4.0-(dq2.*l5.*l6.*m6.*t140)./2.0-(dq3.*l5.*l6.*m6.*t140)./2.0-(dq4.*l5.*l6.*m6.*t140)./2.0-(dq5.*l5.*l6.*m6.*t140)./4.0+(dq2.*l3.*l6.*m6.*t159)./2.0+(dq3.*l3.*l6.*m6.*t159)./2.0+(dq4.*l3.*l6.*m6.*t159)./4.0-(dq5.*l3.*l6.*m6.*t159)./4.0+(dq2.*l5.*l6.*m6.*t217)./2.0+(dq3.*l5.*l6.*m6.*t217)./2.0+(dq4.*l5.*l6.*m6.*t217)./2.0-(dq5.*l5.*l6.*m6.*t217)./4.0;
mt1 = [et1+et2+et3+et4+et5+et6,t99+t100+t101-t130-t135+t152+t153+t154+t155+t179+t212+t255+t262+t270+t271+t283+t285+t286+t288+t291+t292+t293+t294+t310+t311+t320-t339+t348+t353+t372+t374+t377+t388+t389+t392+t393+t394+t396+t397+t407+t409+t411+t412+t413+t418+t419+t420+t422+t424+t427+t433+t435+t437,t96+t97+t98+t147+t162+t169+t170+t171+t179+t255+t262+t270+t271+t275+t283+t285+t286+t289+t291+t292+t293+t294+t298+t310+t311+t320+t348+t353+t372+t374+t376+t377+t388+t389+t392+t393+t394+t396+t397+t407+t409+t411+t412+t413+t418+t419+t420+t422+t424+t427+t433+t435+t437,-t94+t136+t147+t162+t255+t258+t262+t270+t271+t275+t285+t289+t291+t298-t300+t310+t312+t320+t348+t353+t372+t374+t376+t377+t388+t389+t392+t393+t394+t396+t397+t407+t409+t411+t412+t414+t418+t419+t420+t422+t424+t427+t433+t435+t437];
mt2 = [t59+t133+t136+t144+t146+t147+t185-t194-t195+t199+t201+t203+t213+t220+t221+t222+t226+t227+t228+t229+t230+t231+t241+t256+t264+t265+t266+t280+t285+t289+t296+t297+t312-t317-t318-t319+t323+t324+t325+t326+t327+t328+t333+t335+t337+t340-t350-t351-t352+t354+t359+t361+t363+t365+t367+t369+t378+t380+t381+t382+t401+t404+t405+t406+t416+t418+t419+t426+t427+t429+t430+t434+t435,t448];
mt3 = [-t99-t100-t101+t109+t110+t111+t112+t122+t123+t124+t130-t133-t152-t153-t154-t155+t173+t175+t198+t200+t202+t204+t208+t223+t232+t233+t252+t253+t254+t256+t267-t288+t296+t297+t299+t309+t313+t314+t315+t317+t318+t319+t320+t332+t333+t334+t335+t336+t337+t339+t341+t348+t350+t351+t352+t353+t354+t359+t360+t361+t362+t363+t364+t365+t366+t367+t368+t369+t370+t372+t374+t375+t380+t381+t382+t388+t392+t393+t395+t398+t399+t400+t402+t404+t405+t406+t408+t410+t415+t417+t421+t423+t425+t426+t428+t429+t430+t434-dq2.*l2.*l4.*m4.*t2-dq2.*l2.*l4.*m6.*t2];
mt4 = [(dq4.*(t50+t69-t71+t72+t102+t103))./2.0-(dq3.*(-t69+t71-t102-t103+l2.*l3.*m3.*t6.*2.0+l2.*l3.*m4.*t6.*2.0+l2.*l3.*m6.*t6.*2.0))./2.0-(dq5.*(t70+t128+t129+t156+t196+l2.*l6.*m6.*t3.*t4.*t5.*2.0-l2.*l6.*m6.*t5.*t6.*t7.*2.0))./2.0,t55+t56+t57+t58+t79+t82+t113+t114+t160+t161+t184+t240+t248+t249,t79+t84+t85+t113+t115+t116+t160+t161+t184+t240+t248+t249,t121+t132+t134+t137+t143+t145+t186+t187+t188+t189+t190+t191+t197-t209+t211+t214+t219+t224+t225+t234+t235+t236+t263+t272+t273+t274+t278+t295+t321+t322+t331+t344+t355+t357+t379+t384+t403,t447];
mt5 = [-t96-t97-t98+t109+t110+t111+t112+t122+t123+t124+t131-t169-t170-t171+t173+t175+t176+t198+t200+t202+t204+t208+t223+t232+t233+t250+t252+t253+t254+t267+t280+t296+t297+t299+t301+t309+t313+t314+t315+t317+t318+t319+t320+t332+t333+t334+t335+t336+t337+t340+t341+t348+t350+t351+t352+t353+t354+t359+t360+t361+t362+t363+t364+t365+t366+t367+t368+t369+t370+t372+t374+t375+t380+t381+t382+t388+t392+t393+t395+t398+t399+t400+t402+t404+t405+t406+t408+t410+t415+t417+t421+t423+t425+t426+t428+t429+t430+t434,t55-t56-t57-t58+t166+t167+t174+t177+t178+t180+t184+t215-t216+t240+t248+t249+t278+t281+t282-t284-dq3.*l2.*l3.*m3.*t6-dq3.*l2.*l3.*m4.*t6-dq3.*l2.*l3.*m6.*t6+dq2.*l2.*l5.*m6.*t27+dq3.*l2.*l5.*m6.*t27+dq4.*l2.*l5.*m6.*t27];
mt6 = [(dq4.*(t50+t72))./2.0-(dq5.*(t70+t128+t129+t156+t196))./2.0,t84+t85+t115+t116+t184+t240+t248+t249,t121+t134+t137+t143+t186+t187+t188+t189+t190+t191+t197+t211+t214+t219+t224+t225+t234+t235+t236+t263+t272+t273+t274+t295+t321+t322+t331+t344+t355+t357+t379+t384+t403,t447,t94+t122+t123+t124+t131+t164+t176+t198+t200+t202+t204+t213+t223+t232+t233+t250+t252+t253+t254+t267+t280+t299+t300+t301+t309+t317+t318+t319+t320+t332+t333+t334+t335+t336+t337+t340+t342+t348+t350+t351+t352+t353+t354+t359+t360+t361+t362+t363+t364+t365+t366+t367+t368+t369+t370+t372+t374+t375+t380+t381+t382+t388+t392+t393+t395+t398+t399+t401+t402+t404+t405+t406+t408+t410+t415+t417+t421+t423+t425+t426+t428+t429+t430+t434];
mt7 = [t53+t54+t55+t77-t79+t80+t81+t82+t107+t108+t114+t184+t240+t248+t249+dq3.*l2.*l5.*m6.*t3.*t4+dq4.*l2.*l5.*m6.*t3.*t4-dq3.*l2.*l5.*m6.*t6.*t7-dq4.*l2.*l5.*m6.*t6.*t7-dq5.*l2.*l6.*m6.*t3.*t4.*t5+dq3.*l2.*l6.*m6.*t3.*t7.*t8+dq3.*l2.*l6.*m6.*t4.*t6.*t8+dq4.*l2.*l6.*m6.*t3.*t7.*t8+dq4.*l2.*l6.*m6.*t4.*t6.*t8+dq5.*l2.*l6.*m6.*t5.*t6.*t7,t53+t54+t55+t80+t81+t82+t114+t184+t240+t248+t249,(dq5.*t24.*((m5.*t16)./1.2e+1+m6.*t17.*(1.3e+1./1.2e+1)-(m5.*t22)./4.0-(m6.*t22)./4.0))./2.0,t121+t186+t187+t188+t189+t190+t191+t197+t219+t224+t225+t234+t235+t236+t263+t272+t273+t274+t321+t322+t331+t344+t355+t357+t379+t384+t403,t447];
mt8 = [-t59+t135+t150+t164+t176-t185+t194+t195+t198+t200+t202+t204+t205+t212+t220+t221+t222+t226+t227+t228+t229+t230+t231-t241+t258+t264+t265+t266+t283+t298+t299+t301+t303+t305+t307-t309+t310+t317+t318+t319+t342+t345+t346+t347+t350+t351+t352-t359+t360-t361+t362-t363+t364-t365+t366-t367+t368-t369+t370+t376-t378+t385+t386+t387+t389+t414-t416+t421+t422+t423+t424+t425+t428+t433+t437,t60-t132+t142+t163+t165+t166+t167+t172+t174+t177+t178+t180+t181+t182+t183+t209+t216+t237+t238+t239+t242+t243+t244+t245+t246+t247+t251+t257+t259+t260+t261+t268+t269+t276-t278-t281-t282+t284+t290+t302+t316+t343+t349+t356+t358+t383+t390+t391];
mt9 = [t60+t142+t163+t165+t166+t167+t172+t181+t182+t183+t216+t237+t238+t239+t242+t243+t244+t245+t246+t247+t251+t257+t259+t260+t261+t268+t269+t276+t290+t302+t316+t343+t349+t356+t358+t383+t390+t391,t60+t142+t181+t182+t183+t237+t238+t239+t242+t243+t244+t245+t246+t247+t251+t261+t268+t269+t290+t302+t316+t343+t349+t356+t358+t383+t390+t391,0.0,-t117-t118-t119-t431,t448,t446,t446,t446,t117+t118+t119+t431,0.0];
C = reshape([mt1,mt2,mt3,mt4,mt5,mt6,mt7,mt8,mt9],6,6);

== matlab function BS_ur10v/BS control/Cc_v ==
  data: param_noti input; C output; q input; dq input
function C = Cc_v(param_noti, q, dq)
%#codegen
l1 = param_noti(1);
l2 = param_noti(2);
l3 = param_noti(3);
l4 = param_noti(4);
l5 = param_noti(5);
l6 = param_noti(6);
r  = param_noti(7);

m1 = param_noti(8);
m2 = param_noti(9);
m3 = param_noti(10);
m4 = param_noti(11);
m5 = param_noti(12);
m6 = param_noti(13);


q1 = q(1);
q2 = q(2);
q3 = q(3);
q4 = q(4);
q5 = q(5);
q6 = q(6);

qd1 = dq(1);
qd2 = dq(2);
qd3 = dq(3);
qd4 = dq(4);
qd5 = dq(5);
qd6 = dq(6);

%    This function was generated by the Symbolic Math Toolbox version 9.0.
%    01-Oct-2022 22:02:31

t2 = cos(q2);
t3 = cos(q3);
t4 = cos(q4);
t5 = cos(q5);
t6 = sin(q3);
t7 = sin(q4);
t8 = sin(q5);
t9 = q2+q3;
t10 = q2+q5;
t11 = q3+q4;
t12 = q4+q5;
t13 = l2.^2;
t14 = l3.^2;
t15 = l4.^2;
t16 = l5.^2;
t17 = l6.^2;
t18 = q2.*2.0;
t19 = q3.*2.0;
t20 = q4.*2.0;
t21 = q5.*2.0;
t22 = r.^2;
t34 = -q5;
t23 = sin(t18);
t24 = sin(t21);
t25 = l3.*t4;
t26 = cos(t9);
t27 = cos(t10);
t28 = cos(t11);
t29 = cos(t12);
t30 = l3.*t7;
t31 = q4+t9;
t32 = q5+t9;
t33 = q5+t11;
t35 = -t21;
t38 = t9+t12;
t40 = q2+t9;
t45 = l2.*l3.*m3.*t6;
t46 = l2.*l3.*m4.*t6;
t47 = l2.*l3.*m6.*t6;
t48 = l4.*l6.*m6.*t8;
t50 = q2+t34;
t51 = q4+t34;
t52 = t9.*2.0;
t55 = t9+t34;
t56 = t11+t34;
t62 = l2.*l5.*m6.*t3.*t4;
t64 = l2.*l5.*m6.*t6.*t7;
t83 = l2.*l6.*m6.*t3.*t4.*t5;
t84 = l2.*l6.*m6.*t3.*t7.*t8;
t85 = l2.*l6.*m6.*t4.*t6.*t8;
t86 = l2.*l6.*m6.*t5.*t6.*t7;
t105 = (m6.*qd2.*t8.*t22)./4.0;
t106 = (m6.*qd3.*t8.*t22)./4.0;
t107 = (m6.*qd4.*t8.*t22)./4.0;
t108 = (m6.*qd5.*t8.*t22)./4.0;
t109 = (m6.*qd6.*t8.*t22)./4.0;
t118 = (m5.*t5.*t8.*t22)./4.0;
t119 = (m6.*t5.*t8.*t22)./4.0;
t135 = (m5.*t5.*t8.*t16)./1.2e+1;
t157 = m6.*t5.*t8.*t17.*(1.3e+1./1.2e+1);
t36 = cos(t32);
t37 = cos(t33);
t39 = sin(t31);
t41 = q2+t31;
t42 = sin(t40);
t43 = l2.*t28;
t44 = l5.*m6.*t25;
t49 = sin(t38);
t53 = cos(t50);
t54 = cos(t51);
t58 = t12+t32;
t59 = t10+t31;
t60 = l3.*l4.*m4.*t26;
t61 = l3.*l4.*m6.*t26;
t63 = l6.*m6.*t5.*t25;
t65 = l6.*m6.*t8.*t30;
t66 = t9+t31;
t67 = sin(t52);
t68 = cos(t55);
t69 = cos(t56);
t70 = t31+t34;
t71 = t31+t35;
t75 = t45./2.0;
t76 = t46./2.0;
t77 = t47./2.0;
t80 = t9+t38;
t88 = -t62;
t90 = -t64;
t94 = t20+t52;
t97 = t31+t38;
t101 = (l2.*l6.*m6.*t27)./2.0;
t102 = (l3.*l6.*m6.*t29)./4.0;
t110 = -t84;
t111 = -t85;
t112 = -t86;
t113 = t31+t55;
t123 = (m2.*t13.*t23)./2.0;
t124 = (m3.*t13.*t23)./2.0;
t125 = (m4.*t13.*t23)./2.0;
t126 = (m6.*t13.*t23)./2.0;
t127 = -t108;
t128 = -t109;
t131 = t83./2.0;
t134 = t86./2.0;
t136 = -t118;
t137 = -t119;
t139 = t38.*2.0;
t145 = (m5.*t16.*t24)./2.4e+1;
t146 = (m5.*t16.*t24)./4.8e+1;
t147 = (m5.*t22.*t24)./8.0;
t148 = (m6.*t22.*t24)./8.0;
t149 = (m5.*t22.*t24)./1.6e+1;
t150 = (m6.*t22.*t24)./1.6e+1;
t156 = -t135;
t165 = m6.*t17.*t24.*(1.3e+1./2.4e+1);
t166 = m6.*t17.*t24.*(1.3e+1./4.8e+1);
t177 = -t157;
t57 = cos(t41);
t72 = cos(t59);
t73 = sin(t58);
t74 = t44./2.0;
t78 = l4.*l5.*m6.*t39;
t79 = cos(t66);
t81 = sin(t70);
t82 = sin(t71);
t87 = cos(t80);
t89 = -t63;
t91 = l2.*l3.*m3.*t42;
t92 = l2.*l3.*m4.*t42;
t93 = l2.*l3.*m6.*t42;
t95 = t34+t41;
t98 = sin(t94);
t100 = (l5.*m6.*t43)./2.0;
t103 = t63./2.0;
t104 = t25+t43;
t115 = -t102;
t120 = sin(t97);
t121 = (l3.*l6.*m6.*t36)./2.0;
t122 = (l2.*l6.*m6.*t37)./4.0;
t130 = (l6.*m6.*t5.*t43)./2.0;
t132 = (l4.*l6.*m6.*t49)./2.0;
t133 = (l5.*l6.*m6.*t49)./2.0;
t140 = cos(t113);
t151 = sin(t139);
t153 = -t131;
t155 = -t134;
t158 = t34+t94;
t159 = t35+t94;
t160 = (l2.*l6.*m6.*t53)./2.0;
t161 = (l3.*l6.*m6.*t54)./4.0;
t162 = (m5.*t16.*t39)./2.4e+1;
t163 = (m5.*t22.*t39)./8.0;
t164 = (m6.*t22.*t39)./8.0;
t167 = -t147;
t168 = -t148;
t169 = -t149;
t170 = -t150;
t174 = (l3.*l6.*m6.*t68)./2.0;
t175 = (l2.*l6.*m6.*t69)./4.0;
t176 = t44+t65;
t182 = m6.*t17.*t39.*(1.3e+1./2.4e+1);
t183 = (m3.*t14.*t67)./2.0;
t184 = (m4.*t14.*t67)./2.0;
t185 = (m6.*t14.*t67)./2.0;
t279 = t135+t136+t137+t157;
t282 = -qd3.*(t118+t119+t156+t177);
t285 = t45+t46+t47+t64+t88+t110+t111;
t286 = t63+t118+t119+t156+t177;
t96 = l2.*l5.*m6.*t57;
t99 = cos(t95);
t114 = -t100;
t116 = -t103;
t117 = -t81;
t138 = l3.*l5.*m6.*t79;
t141 = t91./2.0;
t142 = t92./2.0;
t143 = t93./2.0;
t144 = -t122;
t154 = -t132;
t171 = sin(t158);
t172 = sin(t159);
t179 = (l2.*l6.*m6.*t72)./2.0;
t180 = (l2.*l6.*m6.*t72)./4.0;
t181 = -t160;
t186 = -t174;
t187 = -t175;
t190 = (l4.*l6.*m6.*t81)./2.0;
t191 = (l5.*l6.*m6.*t81)./2.0;
t192 = t49+t81;
t193 = qd2.*t176;
t194 = qd3.*t176;
t195 = qd4.*t176;
t196 = (m5.*t16.*t73)./4.8e+1;
t197 = (m5.*t22.*t73)./1.6e+1;
t198 = (m6.*t22.*t73)./1.6e+1;
t200 = (l3.*l6.*m6.*t87)./2.0;
t201 = (l3.*l6.*m6.*t87)./4.0;
t202 = (m5.*t16.*t82)./4.8e+1;
t204 = m6.*t17.*t73.*(1.3e+1./4.8e+1);
t205 = (m5.*t22.*t82)./1.6e+1;
t207 = (m6.*t22.*t82)./1.6e+1;
t214 = (l5.*l6.*m6.*t120)./2.0;
t215 = (l5.*l6.*m6.*t120)./4.0;
t216 = (l6.*m6.*t5.*t104)./2.0;
t218 = m6.*t17.*t82.*(1.3e+1./4.8e+1);
t222 = (m6.*t16.*t98)./2.0;
t225 = (l3.*l6.*m6.*t140)./2.0;
t226 = (l3.*l6.*m6.*t140)./4.0;
t230 = (m4.*t15.*t98)./2.4e+1;
t231 = (m5.*t16.*t98)./4.8e+1;
t232 = (m4.*t22.*t98)./8.0;
t233 = (m5.*t22.*t98)./1.6e+1;
t234 = (m6.*t22.*t98)./1.6e+1;
t238 = m6.*t17.*t98.*(1.3e+1./4.8e+1);
t245 = (m5.*t22.*t151)./3.2e+1;
t246 = (m6.*t22.*t151)./3.2e+1;
t248 = (m5.*t16.*t151)./9.6e+1;
t255 = m6.*t17.*t151.*(1.3e+1./9.6e+1);
t278 = t62+t84+t85+t90+t176;
t283 = t145+t165+t167+t168;
t287 = qd2.*t285;
t288 = qd3.*t285;
t289 = qd3.*t286;
t290 = qd5.*t286;
t293 = t83+t112+t286;
t295 = t130+t131+t155+t286;
t296 = t89+t130+t134+t153+t279;
t297 = -qd2.*(-t130+t131+t155+t286);
t129 = -t96;
t152 = t96./2.0;
t178 = -t138;
t188 = t138./2.0;
t189 = -t180;
t199 = -t191;
t203 = -t196;
t206 = -t197;
t208 = -t198;
t209 = (l2.*l6.*m6.*t99)./2.0;
t210 = (l2.*l6.*m6.*t99)./4.0;
t211 = -t201;
t212 = -t194;
t213 = t49+t117;
t217 = -t202;
t219 = -t204;
t220 = -t205;
t221 = -t207;
t227 = -t214;
t228 = -t218;
t229 = -t222;
t235 = -t225;
t236 = -t230;
t237 = -t231;
t239 = -t232;
t240 = -t233;
t241 = -t234;
t242 = (l5.*l6.*m6.*t171)./2.0;
t243 = (l5.*l6.*m6.*t171)./4.0;
t244 = -t238;
t249 = (m5.*t22.*t172)./3.2e+1;
t250 = -t245;
t251 = (m6.*t22.*t172)./3.2e+1;
t252 = -t246;
t253 = (m5.*t16.*t172)./9.6e+1;
t254 = -t248;
t259 = m6.*t17.*t172.*(1.3e+1./9.6e+1);
t260 = -t255;
t261 = (m6.*qd1.*t22.*t192)./8.0;
t262 = (m6.*qd5.*t22.*t192)./8.0;
t263 = (m6.*qd6.*t22.*t192)./8.0;
t280 = qd2.*t278;
t281 = qd4.*t278;
t284 = qd4.*t283;
t291 = -t288;
t292 = -t290;
t294 = qd2.*t293;
t298 = t103+t118+t119+t131+t155+t156+t177+t216;
t299 = t116+t134+t153+t216+t279;
t300 = -qd2.*(t103+t118+t119+t131+t155+t156+t177-t216);
t173 = -t152;
t223 = -t209;
t224 = -t210;
t247 = -t242;
t256 = -t249;
t257 = -t251;
t258 = -t253;
t264 = -t259;
t265 = -t262;
t266 = (m6.*qd1.*t22.*t213)./8.0;
t267 = (m6.*qd2.*t22.*t213)./8.0;
t268 = (m6.*qd3.*t22.*t213)./8.0;
t269 = (m6.*qd4.*t22.*t213)./8.0;
t270 = (m6.*qd6.*t22.*t213)./8.0;
t302 = t78+t133+t154+t190+t191+t197+t198+t202+t203+t218+t219+t220+t221;
t305 = t132+t162+t163+t164+t182+t190+t196+t202+t204+t206+t208+t218+t220+t221;
t306 = t133+t162+t163+t164+t182+t197+t198+t199+t203+t205+t207+t217+t219+t228;
t271 = -t266;
t272 = -t267;
t273 = -t268;
t274 = -t269;
t275 = -t270;
t276 = t127+t266;
t303 = qd4.*t302;
t307 = qd5.*t305;
t308 = qd1.*t306;
t309 = t60+t61+t121+t174+t302;
t311 = t121+t186+t306;
t316 = t48+t102+t122+t146+t161+t166+t169+t170+t175+t180+t201+t210+t215+t226+t243+t245+t246+t253+t254+t256+t257+t259+t260;
t318 = t74+t100+t115+t144+t152+t161+t175+t188+t189+t210+t211+t222+t226+t227+t230+t233+t234+t237+t239+t242+t244+t248+t250+t252+t253+t255+t256+t257+t259;
t320 = t91+t92+t93+t123+t124+t125+t126+t129+t178+t179+t183+t184+t185+t200+t214+t223+t229+t231+t232+t235+t236+t238+t240+t241+t245+t246+t247+t249+t251+t254+t258+t260+t264;
t322 = t75+t76+t77+t114+t122+t141+t142+t143+t173+t178+t180+t183+t184+t185+t187+t200+t214+t224+t229+t231+t232+t235+t236+t238+t240+t241+t245+t246+t247+t249+t251+t254+t258+t260+t264;
t277 = t127+t271;
t301 = t265+t272+t273+t274;
t304 = -t303;
t310 = qd3.*t309;
t313 = qd1.*t311;
t314 = t101+t181+t311;
t317 = qd1.*t316;
t319 = qd1.*t318;
t321 = qd1.*t320;
t323 = qd1.*t322;
t312 = -t310;
t315 = qd1.*t314;
mt1 = [-qd5.*t316-qd2.*t320+qd4.*t318-qd3.*t322,t270+t321-qd5.*t314,t270+t323-qd5.*t311,t270-t319-qd5.*t306,t263+t317+qd4.*t306+qd3.*t311+qd2.*t314,t301,t275+t304+t307+t312-t321-qd2.*(t101+t160+t309+l2.*l4.*m4.*t2+l2.*l4.*m6.*t2),t281+t291-qd5.*t293,t195+t287-qd5.*(-t130+t131+t155+t286),t212-t280-qd5.*(t103+t118+t119+t131+t155+t156+t177-t216),t109+t294+t315+qd4.*(t103+t118+t119+t131+t155+t156+t177-t216)+qd3.*(-t130+t131+t155+t286),t277,t275+t304+t307+t312-t323-qd2.*t309,t281-t287+t291-qd5.*t295,t195+t292];
mt2 = [-t193+t212-qd5.*(t118+t119+t156+t177),t109+t289+t313+qd4.*(t118+t119+t156+t177)+qd2.*(-t130+t131+t155+t286),t277,t275+t304+t307+t319-qd2.*t302-qd3.*t302,t280+t281+qd3.*t278-qd5.*t298,t193+t194+t195+t292,qd5.*t283,t109-t284+t308+qd3.*(t118+t119+t156+t177)+qd2.*(t103+t118+t119+t131+t155+t156+t177-t216),t277,-t263-t317+qd5.*(t101+t121+t132+t133+t160+t174-t190+t191)+qd2.*t305+qd3.*t305+qd4.*t305,t128-t294-t315-qd3.*t295-qd4.*t298+l6.*m6.*qd5.*t8.*(l5+t30+l2.*sin(t11)),t128-t289+t297-t313-qd4.*t286+l6.*m6.*qd5.*t8.*(l5+t30)];
mt3 = [t128+t282+t284+t300-t308+l5.*l6.*m6.*qd5.*t8,0.0,-t105-t106-t107-t261,t301,t276,t276,t276,t105+t106+t107+t261,0.0];
C = reshape([mt1,mt2,mt3],6,6);

== matlab function BS_ur10v/Ur10 dynamics/G_v ==
  data: param_noti input; G output; q input
function G = G_v(param_noti, q)
%#codegen

l1 = param_noti(1);
l2 = param_noti(2);
l3 = param_noti(3);
l4 = param_noti(4);
l5 = param_noti(5);
l6 = param_noti(6);
r  = param_noti(7);

m1 = param_noti(8);
m2 = param_noti(9);
m3 = param_noti(10);
m4 = param_noti(11);
m5 = param_noti(12);
m6 = param_noti(13);


q1 = q(1);
q2 = q(2);
q3 = q(3);
q4 = q(4);
q5 = q(5);
q6 = q(6);
%    This function was generated by the Symbolic Math Toolbox version 9.0.
%    24-Sep-2022 17:50:00

t2 = cos(q2);
t3 = q2+q3;
t6 = -q5;
t4 = cos(t3);
t5 = q4+t3;
t7 = q5+t5;
t8 = sin(t5);
t10 = t5+t6;
t12 = l3.*m3.*t4.*(9.81e+2./1.0e+2);
t13 = l3.*m4.*t4.*(9.81e+2./1.0e+2);
t14 = l3.*m6.*t4.*(9.81e+2./1.0e+2);
t9 = sin(t7);
t11 = sin(t10);
t15 = l5.*m6.*t8.*(9.81e+2./1.0e+2);
t16 = -t12;
t17 = -t13;
t18 = -t14;
t19 = -t15;
t20 = l6.*m6.*t9.*(9.81e+2./2.0e+2);
t21 = l6.*m6.*t11.*(9.81e+2./2.0e+2);
t22 = -t21;
G = [0.0;t16+t17+t18+t19+t20+t22-l2.*m2.*t2.*(9.81e+2./1.0e+2)-l2.*m3.*t2.*(9.81e+2./1.0e+2)-l2.*m4.*t2.*(9.81e+2./1.0e+2)-l2.*m6.*t2.*(9.81e+2./1.0e+2);t16+t17+t18+t19+t20+t22;m6.*(l5.*t8-(l6.*t9)./2.0+(l6.*t11)./2.0).*(-9.81e+2./1.0e+2);l6.*m6.*(t9+t11).*(9.81e+2./2.0e+2);0.0];

== matlab function BS_ur10v/BS control/B_v ==
  data: param_noti input; B output; q input
function B = B_v(param_noti, q)

l1 = param_noti(1);
l2 = param_noti(2);
l3 = param_noti(3);
l4 = param_noti(4);
l5 = param_noti(5);
l6 = param_noti(6);
r  = param_noti(7);

m1 = param_noti(8);
m2 = param_noti(9);
m3 = param_noti(10);
m4 = param_noti(11);
m5 = param_noti(12);
m6 = param_noti(13);

q1 = q(1);
q2 = q(2);
q3 = q(3);
q4 = q(4);
q5 = q(5);
q6 = q(6);
%#codegen

%    This function was generated by the Symbolic Math Toolbox version 9.0.
%    24-Sep-2022 17:40:10

t2 = cos(q3);
t3 = cos(q4);
t4 = cos(q5);
t5 = sin(q2);
t6 = sin(q3);
t7 = sin(q4);
t8 = sin(q5);
t9 = q2+q3;
t10 = q2+q5;
t11 = q3+q4;
t12 = l2.^2;
t13 = l3.^2;
t14 = l4.^2;
t15 = l5.^2;
t16 = l6.^2;
t17 = q2.*2.0;
t18 = q3.*2.0;
t19 = q4.*2.0;
t20 = q5.*2.0;
t21 = r.^2;
t31 = -q5;
t22 = cos(t17);
t23 = cos(t20);
t24 = t4.^2;
t25 = l3.*t7;
t26 = q4+t9;
t27 = q5+t9;
t28 = sin(t9);
t29 = sin(t10);
t30 = sin(t11);
t32 = -t20;
t36 = m3.*t13;
t37 = m4.*t13;
t38 = m6.*t13;
t39 = m6.*t15;
t40 = q2+t9;
t42 = l2.*l3.*m3.*t2;
t43 = l2.*l3.*m4.*t2;
t44 = l2.*l3.*m6.*t2;
t45 = l5.*l6.*m6.*t4;
t49 = l2.*l4.*m4.*t5;
t50 = l2.*l4.*m6.*t5;
t52 = q2+t31;
t53 = t9.*2.0;
t54 = t9+t31;
t60 = l2.*l5.*m6.*t2.*t7;
t61 = l2.*l5.*m6.*t3.*t6;
t62 = l3.*l6.*m6.*t3.*t8;
t70 = (m3.*t21)./2.0;
t71 = (m4.*t21)./4.0;
t72 = (m5.*t21)./4.0;
t73 = (m6.*t21)./4.0;
t76 = (m4.*t14)./1.2e+1;
t77 = (m5.*t15)./1.2e+1;
t81 = l2.*l6.*m6.*t2.*t3.*t8;
t82 = l2.*l6.*m6.*t6.*t7.*t8;
t87 = (m6.*t4.*t21)./2.0;
t88 = m6.*t16.*(1.3e+1./1.2e+1);
t33 = cos(t26);
t34 = q5+t26;
t35 = sin(t27);
t41 = cos(t40);
t46 = l5+t25;
t47 = l2.*t30;
t51 = l5.*m6.*t25;
t55 = sin(t52);
t56 = t20+t26;
t58 = l3.*l4.*m4.*t28;
t59 = l3.*l4.*m6.*t28;
t63 = cos(t53);
t64 = -t45;
t65 = t26+t31;
t66 = t26+t32;
t67 = sin(t54);
t68 = -t49;
t69 = -t50;
t75 = t62.*2.0;
t85 = -t62;
t89 = t19+t53;
t91 = (l2.*l6.*m6.*t29)./2.0;
t93 = -t81;
t97 = t24.*t72;
t98 = t24.*t73;
t107 = t24.*t77;
t116 = m5.*t15.*t24.*(-1.0./1.2e+1);
t117 = t24.*t88;
t123 = m6.*t16.*t24.*(-1.3e+1./1.2e+1);
t48 = cos(t34);
t57 = t51.*2.0;
t74 = cos(t56);
t78 = l4.*l5.*m6.*t33;
t79 = cos(t65);
t80 = cos(t66);
t83 = -t58;
t84 = -t59;
t86 = -t75;
t90 = cos(t89);
t92 = l6.*m6.*t4.*t46;
t95 = -t91;
t96 = (l3.*l6.*m6.*t35)./2.0;
t99 = t46+t47;
t103 = t20+t89;
t104 = t33.*t72;
t105 = t33.*t73;
t111 = t32+t89;
t112 = t33.*t77;
t113 = m5.*t21.*t33.*(-1.0./4.0);
t114 = m6.*t21.*t33.*(-1.0./4.0);
t115 = (l2.*l6.*m6.*t55)./2.0;
t119 = (l3.*l6.*m6.*t67)./2.0;
t120 = m5.*t15.*t33.*(-1.0./1.2e+1);
t121 = t33.*t88;
t127 = m6.*t16.*t33.*(-1.3e+1./1.2e+1);
t145 = t39+t51+t71+t72+t73+t76+t77+t85+t88+t97+t98+t116+t123;
t94 = -t79;
t100 = (l4.*l6.*m6.*t48)./2.0;
t101 = (l5.*l6.*m6.*t48)./2.0;
t102 = -t92;
t106 = -t96;
t108 = cos(t103);
t118 = cos(t111);
t122 = -t115;
t124 = -t119;
t125 = (l4.*l6.*m6.*t79)./2.0;
t126 = (l5.*l6.*m6.*t79)./2.0;
t128 = l6.*m6.*t4.*t99;
t129 = (m5.*t15.*t74)./4.8e+1;
t130 = (m5.*t21.*t74)./1.6e+1;
t131 = (m6.*t21.*t74)./1.6e+1;
t133 = (m5.*t15.*t80)./4.8e+1;
t135 = m6.*t16.*t74.*(1.3e+1./4.8e+1);
t136 = (m5.*t21.*t80)./1.6e+1;
t137 = (m6.*t21.*t80)./1.6e+1;
t140 = m6.*t16.*t80.*(1.3e+1./4.8e+1);
t146 = t60+t61+t82+t93+t145;
t148 = t36+t37+t38+t39+t42+t43+t44+t57+t60+t61+t70+t71+t72+t73+t76+t77+t82+t86+t88+t93+t97+t98+t116+t123;
t109 = -t100;
t110 = -t101;
t132 = -t125;
t134 = -t129;
t138 = -t128;
t139 = t48+t94;
t141 = -t135;
t142 = -t136;
t143 = -t137;
t144 = t73.*t139;
t147 = t91+t96+t109+t110+t113+t114+t120+t122+t124+t126+t127+t132;
t149 = t78+t101+t109+t125+t126+t130+t131+t133+t134+t140+t141+t142+t143;
t150 = t83+t84+t106+t124+t149;
t151 = t68+t69+t95+t122+t150;
et1 = t36.*(7.0./1.2e+1)+t37./2.0+t38./2.0+t39./2.0+t42+t43+t44+t51+m2.*t12.*(7.0./1.2e+1)+(m3.*t12)./2.0+(m4.*t12)./2.0+m4.*t14.*(2.5e+1./2.4e+1)+(m6.*t12)./2.0+(m5.*t15)./1.6e+1+m6.*t14+(m1.*t21)./4.0+m6.*t16.*(1.3e+1./1.6e+1)+(m2.*t21)./4.0+(m3.*t21)./4.0+m4.*t21.*(3.0./8.0)+m5.*t21.*(5.0./1.6e+1)+m6.*t21.*(5.0./1.6e+1)+(t36.*t63)./2.0+(t37.*t63)./2.0+(t38.*t63)./2.0-(t39.*t90)./2.0+(l1.^2.*m1)./1.2e+1+l5.*m6.*t47+(m2.*t12.*t22)./2.0+(m3.*t12.*t22)./2.0+(m4.*t12.*t22)./2.0+(m6.*t12.*t22)./2.0+(m5.*t15.*t23)./4.8e+1+m6.*t16.*t23.*(1.3e+1./4.8e+1);
et2 = m5.*t21.*t23.*(-1.0./1.6e+1)-(m6.*t21.*t23)./1.6e+1-(m4.*t14.*t90)./2.4e+1+(m5.*t15.*t90)./4.8e+1+m6.*t16.*t90.*(1.3e+1./4.8e+1)+(m4.*t21.*t90)./8.0-(m5.*t21.*t90)./1.6e+1-(m6.*t21.*t90)./1.6e+1-(m5.*t15.*t108)./9.6e+1-m6.*t16.*t108.*(1.3e+1./9.6e+1)+(m5.*t21.*t108)./3.2e+1+(m6.*t21.*t108)./3.2e+1-(m5.*t15.*t118)./9.6e+1-m6.*t16.*t118.*(1.3e+1./9.6e+1)+(m5.*t21.*t118)./3.2e+1+(m6.*t21.*t118)./3.2e+1+l4.*l6.*m6.*t4.*2.0+l2.*l3.*m3.*t41+l2.*l3.*m4.*t41+l2.*l3.*m6.*t41-(l5.*l6.*m6.*cos(t31+t89))./2.0-(l3.*l6.*m6.*sin(q4+q5))./2.0;
et3 = l2.*l6.*m6.*sin(q5+t11).*(-1.0./2.0)+l2.*l5.*m6.*sin(q2+t26)+(l3.*l6.*m6.*sin(q4+t31))./2.0+l3.*l5.*m6.*sin(t9+t26)-(l2.*l6.*m6.*sin(t10+t26))./2.0+(l2.*l6.*m6.*sin(t11+t31))./2.0-(l3.*l6.*m6.*sin(t26+t27))./2.0+(l2.*l6.*m6.*sin(t26+t52))./2.0+(l3.*l6.*m6.*sin(t26+t54))./2.0+(l5.*l6.*m6.*cos(t9+t19+t27))./2.0;
B = reshape([et1+et2+et3,t151,t150,t149,t147,t144,t151,t36+t37+t38+t39+t42.*2.0+t43.*2.0+t44.*2.0+t57+t60.*2.0+t61.*2.0+t70+t71+t72+t73+t76+t77-t81.*2.0+t82.*2.0+t86+t88+t97+t98+t116+t123+m2.*t12+m3.*t12+m4.*t12+m6.*t12+(m2.*t21)./2.0,t148,t146,t138,t87,t150,t148,t36+t37+t38+t39+t57+t70+t71+t72+t73+t76+t77+t86+t88+t97+t98+t116+t123,t145,t102,t87,t149,t146,t145,t39+t71+t76+(m5.*t15)./2.4e+1+m6.*t16.*(1.3e+1./2.4e+1)+m5.*t21.*(3.0./8.0)+m6.*t21.*(3.0./8.0)-(m5.*t15.*t23)./2.4e+1-m6.*t16.*t23.*(1.3e+1./2.4e+1)+(m5.*t21.*t23)./8.0+(m6.*t21.*t23)./8.0,t64,t87,t147,t138,t102,t64,t72+t73+t77+t88,0.0,t144,t87,t87,t87,0.0,(m6.*t21)./2.0],[6,6]);
